simulink model "threephase_Inverter"  (R2023a)
settings: Solver=ode23tb  StartTime=0.0  StopTime=1  MaxStep=1e-4  RelTol=1e-3
libraries: spsMosfetLib x12, spsSeriesRLCBranchLib x6, spsThreePhaseVIMeasurementLib x4, spsDCVoltageSourceLib x2, spsGroundLib x2, sps_lib x1
settings Model: Creator=gaming3  LastModifiedBy=gaming3

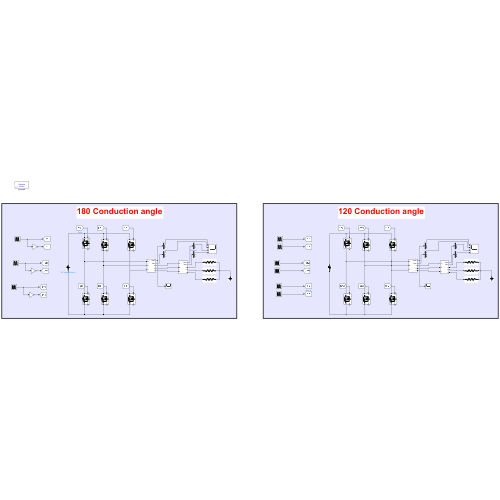
[thumbnail: Simulink's stored preview of the top-level diagram]
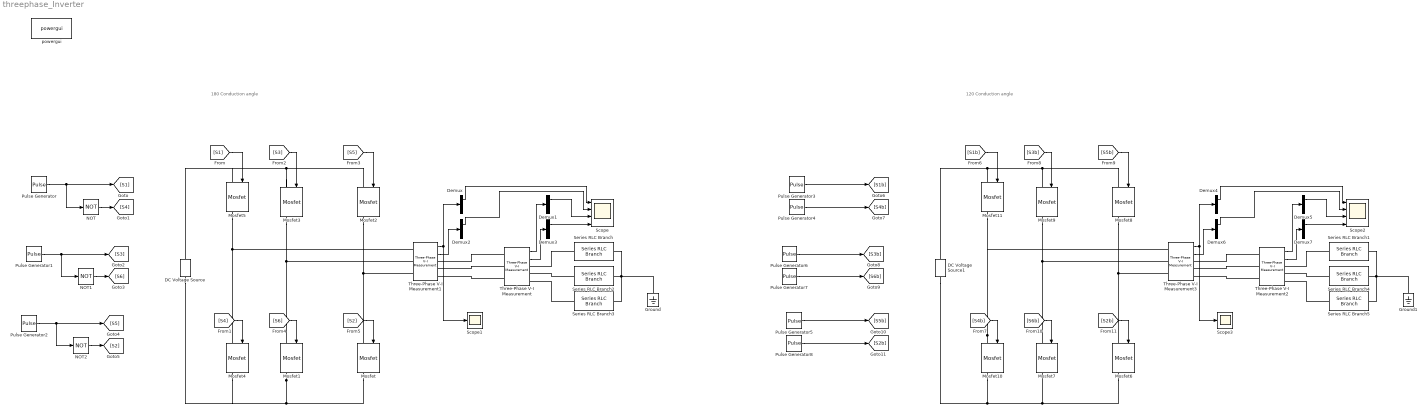
== system threephase_Inverter ==
  note: 180 Conduction angle
  note: 120 Conduction angle
  DC Voltage Source : spsDCVoltageSourceLib/DC Voltage Source  Amplitude=310  Measurements=None
  DC Voltage Source1 : spsDCVoltageSourceLib/DC Voltage Source  Amplitude=310  Measurements=None
  Demux{,1..7} (8 alike) : Demux  Outputs=3
  Ground : spsGroundLib/Ground  LConnTagsString=a
  Ground1 : spsGroundLib/Ground  LConnTagsString=a
  Mosfet{,1..11} (12 alike) : spsMosfetLib/Mosfet  Ron=0.1  Lon=0  Rd=0.01  Vfd=0  IC=0  Rs=1e5  Cs=inf  Measurements=on
  NOT : Logic  Operator=NOT  IconShape=distinctive  AllPortsSameDT=off  OutDataTypeStr=boolean
  NOT1 : Logic  Operator=NOT  IconShape=distinctive  AllPortsSameDT=off  OutDataTypeStr=boolean
  NOT2 : Logic  Operator=NOT  IconShape=distinctive  AllPortsSameDT=off  OutDataTypeStr=boolean
  Pulse Generator : DiscretePulseGenerator  PulseType=Time based  Period=0.02  PulseWidth=50
  Pulse Generator1 : DiscretePulseGenerator  PulseType=Time based  Period=0.02  PulseWidth=50  PhaseDelay=(120*0.02)/360
  Pulse Generator2 : DiscretePulseGenerator  PulseType=Time based  Period=0.02  PulseWidth=50  PhaseDelay=(240*0.02)/360
  Pulse Generator3 : DiscretePulseGenerator  PulseType=Time based  Period=0.02  PulseWidth=100/3
  Pulse Generator4 : DiscretePulseGenerator  PulseType=Time based  Period=0.02  PulseWidth=100/3  PhaseDelay=(180*0.02)/360
  Pulse Generator5 : DiscretePulseGenerator  PulseType=Time based  Period=0.02  PulseWidth=100/3  PhaseDelay=(240*0.02)/360
  Pulse Generator6 : DiscretePulseGenerator  PulseType=Time based  Period=0.02  PulseWidth=100/3  PhaseDelay=(120*0.02)/360
  Pulse Generator7 : DiscretePulseGenerator  PulseType=Time based  Period=0.02  PulseWidth=100/3  PhaseDelay=(300*0.02)/360
  Pulse Generator8 : DiscretePulseGenerator  PulseType=Time based  Period=0.02  PulseWidth=100/3  PhaseDelay=(60*0.02)/360
  Scope : Scope  NumInputPorts=4
  Scope1 : Scope
  Scope2 : Scope  NumInputPorts=4
  Scope3 : Scope
  Series RLC Branch{,1..5} (6 alike) : spsSeriesRLCBranchLib/Series RLC Branch  LConnTagsString=__new0  RConnTagsString=__new0  BranchType=R  Resistance=10  Inductance=1e-3  SetiL0=off  InitialCurrent=0  Capacitance=1e-6  Setx0=off  InitialVoltage=0  Measurements=None
  Three-Phase V-I Measurement : spsThreePhaseVIMeasurementLib/Three-Phase V-I Measurement  VoltageMeasurement=phase-to-phase  SetLabelV=off  LabelV=Vabc  Vpu=off  VpuLL=off  CurrentMeasurement=yes  SetLabelI=off  LabelI=Iabc  Ipu=off  Pbase=100e6  Vbase=500e3  OutputType=Complex  PhasorSimulation=off  PSBequivalent=0
  Three-Phase V-I Measurement1 : spsThreePhaseVIMeasurementLib/Three-Phase V-I Measurement  VoltageMeasurement=phase-to-ground  SetLabelV=off  LabelV=Vabc  Vpu=off  VpuLL=off  CurrentMeasurement=yes  SetLabelI=off  LabelI=Iabc  Ipu=off  Pbase=100e6  Vbase=500e3  OutputType=Complex  PhasorSimulation=off  PSBequivalent=0
  Three-Phase V-I Measurement2 : spsThreePhaseVIMeasurementLib/Three-Phase V-I Measurement  VoltageMeasurement=phase-to-phase  SetLabelV=off  LabelV=Vabc  Vpu=off  VpuLL=off  CurrentMeasurement=yes  SetLabelI=off  LabelI=Iabc  Ipu=off  Pbase=100e6  Vbase=500e3  OutputType=Complex  PhasorSimulation=off  PSBequivalent=0
  Three-Phase V-I Measurement3 : spsThreePhaseVIMeasurementLib/Three-Phase V-I Measurement  VoltageMeasurement=phase-to-ground  SetLabelV=off  LabelV=Vabc  Vpu=off  VpuLL=off  CurrentMeasurement=yes  SetLabelI=off  LabelI=Iabc  Ipu=off  Pbase=100e6  Vbase=500e3  OutputType=Complex  PhasorSimulation=off  PSBequivalent=0
  powergui : sps_lib/powergui  Priority=1  SimulationMode=Discrete  SampleTime=1e-06  frequency=60  Iterations=50  frequencyindice=0  Pbase=100e6  ErrMax=1e-4  UnitsV=kV  UnitsW=MW  buscounter=0  FunctionMessages=off  echomessages=off  EnableUseOfTLC=off  CurrentSourceSwitches=off  DisableSnubberDevices=off  DisableRonSwitches=off  DisableVfSwitches=off  DisplayEquations=off  AutomaticDiscreteSolvers=off  SolverType=Tustin/Backward Euler (TBE)  Interpol=off  ExternalGateDelay=off  methode=off  Ts=100  x0status=blocks  SPID=on  SwTol=0  HookPort=off  NonlinearTolerance=1e-4  nMaxIteration=100  ContinueOnMaxIteration=off  RestoreLinks=warning  ResistiveCurrentMeasurement=off  Frange=[0:2:500]  Ylog=off  Xlog=on  ShowGrid=off  save=off  variable=ZData  structure=0  ZoomFFT=off  StartTime=0.0  cycles=1  DisplayStyle=1  fundamental=60  FreqAxis=off  MaxFrequency=1000  frequencyindicesteady=1  RmsSteady=1  display=off
  wires:
  Pulse Generator/1 -> NOT/1, [S1]
  NOT/1 -> [S4]
  [S1] -> Mosfet5/1
  [S4] -> Mosfet4/1
  NOT1/1 -> [S6]
  Pulse Generator1/1 -> [S3], NOT1/1
  Pulse Generator2/1 -> NOT2/1, [S5]
  NOT2/1 -> [S2]
  [S3] -> Mosfet3/1
  [S5] -> Mosfet2/1
  [S2] -> Mosfet/1
  [S6] -> Mosfet1/1
  Three-Phase V-I Measurement1/1 -> Demux/1, Scope1/1
  Three-Phase V-I Measurement1/2 -> Demux2/1
  Three-Phase V-I Measurement/1 -> Demux1/1
  Three-Phase V-I Measurement/2 -> Demux3/1
  Demux/1 -> Scope/1
  Demux2/1 -> Scope/2
  Demux1/1 -> Scope/3
  Demux3/1 -> Scope/4
  Demux7/1 -> Scope2/4
  Demux5/1 -> Scope2/3
  Demux6/1 -> Scope2/2
  Demux4/1 -> Scope2/1
  Three-Phase V-I Measurement2/2 -> Demux7/1
  Three-Phase V-I Measurement2/1 -> Demux5/1
  Three-Phase V-I Measurement3/2 -> Demux6/1
  Three-Phase V-I Measurement3/1 -> Scope3/1, Demux4/1
  [S6b] -> Mosfet7/1
  [S2b] -> Mosfet6/1
  [S5b] -> Mosfet8/1
  [S3b] -> Mosfet9/1
  Pulse Generator5/1 -> [S5b]
  Pulse Generator6/1 -> [S3b]
  Pulse Generator7/1 -> [S6b]
  [S4b] -> Mosfet10/1
  [S1b] -> Mosfet11/1
  Pulse Generator4/1 -> [S4b]
  Pulse Generator3/1 -> [S1b]
  Pulse Generator8/1 -> [S2b]
  connections:
  Mosfet3/LConn1 -- DC Voltage Source/RConn1 -- Mosfet5/LConn1 -- Mosfet2/LConn1
  Mosfet1/RConn1 -- Mosfet/RConn1 -- Mosfet4/RConn1 -- DC Voltage Source/LConn1
  Mosfet3/RConn1 -- Three-Phase V-I Measurement1/LConn2 -- Mosfet1/LConn1
  Mosfet2/RConn1 -- Three-Phase V-I Measurement1/LConn3 -- Mosfet/LConn1
  Mosfet5/RConn1 -- Mosfet4/LConn1 -- Three-Phase V-I Measurement1/LConn1
  Series RLC Branch/LConn1 -- Ground/LConn1 -- Series RLC Branch2/LConn1 -- Series RLC Branch3/LConn1
  Series RLC Branch/RConn1 -- Three-Phase V-I Measurement/RConn1
  Series RLC Branch2/RConn1 -- Three-Phase V-I Measurement/RConn2
  Series RLC Branch3/RConn1 -- Three-Phase V-I Measurement/RConn3
  Three-Phase V-I Measurement/LConn1 -- Three-Phase V-I Measurement1/RConn1
  Three-Phase V-I Measurement/LConn2 -- Three-Phase V-I Measurement1/RConn2
  Three-Phase V-I Measurement/LConn3 -- Three-Phase V-I Measurement1/RConn3
  DC Voltage Source1/RConn1 -- Mosfet11/LConn1 -- Mosfet9/LConn1 -- Mosfet8/LConn1
  Mosfet10/RConn1 -- DC Voltage Source1/LConn1 -- Mosfet7/RConn1 -- Mosfet6/RConn1
  Three-Phase V-I Measurement3/LConn2 -- Mosfet9/RConn1 -- Mosfet7/LConn1
  Three-Phase V-I Measurement3/LConn3 -- Mosfet8/RConn1 -- Mosfet6/LConn1
  Mosfet10/LConn1 -- Mosfet11/RConn1 -- Three-Phase V-I Measurement3/LConn1
  Ground1/LConn1 -- Series RLC Branch1/LConn1 -- Series RLC Branch5/LConn1 -- Series RLC Branch4/LConn1
  Three-Phase V-I Measurement2/LConn3 -- Three-Phase V-I Measurement3/RConn3
  Three-Phase V-I Measurement2/LConn2 -- Three-Phase V-I Measurement3/RConn2
  Three-Phase V-I Measurement2/LConn1 -- Three-Phase V-I Measurement3/RConn1
  Series RLC Branch5/RConn1 -- Three-Phase V-I Measurement2/RConn3
  Series RLC Branch1/RConn1 -- Three-Phase V-I Measurement2/RConn1
  Series RLC Branch4/RConn1 -- Three-Phase V-I Measurement2/RConn2
